simulink library "fbklib"  (R2015a)
settings: Solver=ode45  SolverMode=SingleTasking  StartTime=0.0  StopTime=10.0  RelTol=1e-3
settings Model: Creator=Fares  LastModifiedBy=Fares
settings DataIOCC: SignalLoggingSaveFormat=ModelDataLogs
settings OptimizationCC: BlockReduction=off  BooleanDataType=off
settings DebuggingCC: SaveWithParameterizedLinksMsg=none  UnderspecifiedInitializationDetection=Classic  MergeDetectMultiDrivingBlocksExec=none  SignalResolutionControl=TryResolveAllWithWarning  MultiTaskDSMMsg=warning  MultiTaskCondExecSysMsg=none  StrictBusMsg=None
settings HardwareCC: TargetUnknown=on

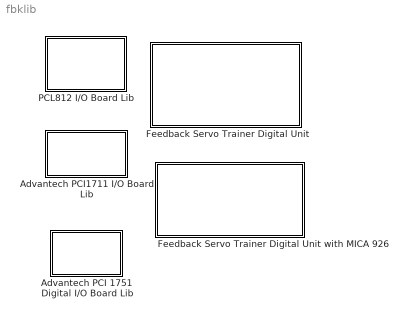
== system fbklib ==
  "Advantech PCI 1751 Digital I/O Board Lib " : Subsystem  AncestorBlock=|  mask(Advantech PCI 1751 Digital I/O Borad Lib.){}
      | pci1751/Advantech 
      | PCI 1751 Digital I//O
      | Board Lib
      mask Display: plot(0,0,100,100,[90,80,80,11,11],[90,90,20,20,80],[11,80],[80,80],[80,80],[20,14],[80,85,85,80],[45,45,66,66],[45,45,74,74],[20,13,13,20],[15,27,27,15,15],[75,75,26,26,75],[33,48,48,33,33],[75,75,55,55,75],[55,55,71,71,55],[55,75,75,55,55],[33,41,41,33,33],[50,50,27,27,50],[48,56,56,48,48],[50,50,27,27,50],[62,70,70,62,62],[50,50,27,27,50])
  Advantech PCI1711 I/O Board Lib : Subsystem  AncestorBlock="pci1711/Advantech  PCI1711 I//O Board Lib"  mask(PCI 1711 I/O Board Lib){}
      mask Display: plot(0,0,100,100,[90,80,80,11,11],[90,90,20,20,80],[11,80],[80,80],[80,80],[20,14],[80,85,85,80],[45,45,66,66],[45,45,74,74],[20,13,13,20],[15,27,27,15,15],[75,75,26,26,75],[33,48,48,33,33],[75,75,55,55,75],[55,55,71,71,55],[55,75,75,55,55],[33,41,41,33,33],[50,50,27,27,50],[48,56,56,48,48],[50,50,27,27,50],[62,70,70,62,62],[50,50,27,27,50])
  Feedback Servo Trainer Digital Unit : Subsystem  AncestorBlock=ServoTrainer/Feedback Servo Trainer Digital Unit  mask(Feedback Servo Trainer Digital Unit){}
      mask Display: disp ('Feedback 33-003 \n\n Digital Servo Fundementals ')
  Feedback Servo Trainer Digital Unit with MICA 926 : Subsystem  AncestorBlock=MicaServo/Feedback Servo Trainer Digital Unit  mask(Feedback Servo Trainer Digital Unit with Mica926){}
      mask Display: disp ('Feedback 33-003 \n\n Digital Servo Fundementals \n with MICA 926')
  PCL812 I/O Board Lib : Subsystem  AncestorBlock=Pcl812fbk/PCL812 I//O Board Lib  mask(PCL812 I/O Board Lib){}
      mask Display: plot(0,0,100,100,[90,80,80,11,11],[90,90,20,20,80],[11,80],[80,80],[80,80],[20,14],[80,85,85,80],[45,45,66,66],[45,45,74,74],[20,13,13,20],[15,27,27,15,15],[75,75,26,26,75],[33,48,48,33,33],[75,75,55,55,75],[55,55,71,71,55],[55,75,75,55,55],[33,41,41,33,33],[50,50,27,27,50],[48,56,56,48,48],[50,50,27,27,50],[62,70,70,62,62],[50,50,27,27,50])

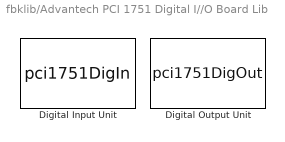
== system fbklib/Advantech PCI 1751 Digital I//O Board Lib  ==
  Digital Input Unit : S-Function  FunctionName=pci1751DigIn  Parameters=channel,portName,tsamp,hwaccess  mask(Digital Input Unit){channel=0, portName=A, tsamp=0.001, hwaccess=on}
      mask prompts: channel "Channel (0 or 1)"; portName "Input Port (A, B or  C)"; tsamp "sample Time (sec)"; hwaccess "Access Hardware"
      mask help: Digital Input Block for PCI1751
      mask Display: disp('PCI1751 \n Lab I/O Board \n\n Digital Input')
  Digital Output Unit : S-Function  FunctionName=pci1751DigOut  Parameters=channel,portName,tsamp,hwaccess  mask(Digital Output Unit){channel=0, portName=A, tsamp=0.001, hwaccess=on}
      mask prompts: channel "Channel (0 or 1)"; portName "Output Port (A, B, C or D)"; tsamp "sample Time (sec)"; hwaccess "Access Hardware"
      mask help: DigitalOutput Block for PCI1751
      mask Display: disp('PCI1751 \n Lab I/O Board \n\n Digital Output')

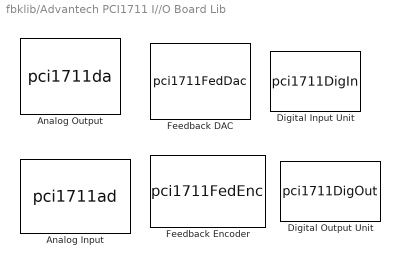
== system fbklib/Advantech PCI1711 I//O Board Lib ==
  Analog Input : S-Function  FunctionName=pci1711ad  Parameters=channel,rangeGain,tsamp,hwAccess  mask(Analog Input Unit){channel=0, rangeGain=0, tsamp=0.001, hwAccess=on}
      mask prompts: channel "Input Channel"; rangeGain "ADC Range Gain  (0 for -/+5V 1 for -/+2.5V 2 for -/+1.25 3 for -/+0.625V)"; tsamp "sampling Time (sec)"; hwAccess "Hardware Access"
      mask help:
      | Analog to Digital Input block for the
      |  Advantech PCI1711  I/O board
      mask Display: disp('PCI1711\n Lab I/O Board \n\n ADC')
  Analog Output : S-Function  FunctionName=pci1711da  Parameters=outChannel,range,tsamp,hwAccess  mask(Analog Output Unit){outChannel=0, range=0, tsamp=0.001, hwAccess=on}
      mask prompts: outChannel "Output Channel"; range "Range Selector (0 for 0-5V and 1 for 0-10V range)"; tsamp "sample Time (sec)"; hwAccess "Access Hardware"
      mask help:
      | Digital to Analog Output block for the
      |  Advantech PCI1711  I/O board
      mask Display: disp('PCI1711 \n Lab I/O Board \n\n DAC')
  Digital Input Unit : S-Function  FunctionName=pci1711DigIn  Parameters=channel,tsamp,hwaccess  mask(Digital Input Unit){channel=0, tsamp=0.001, hwaccess=on}
      mask prompts: channel "Channel (0 or 1)"; tsamp "sample Time (sec)"; hwaccess "Access Hardware"
      mask help: Digital Input Block
      mask Display: disp('PCI1711 \n Lab I/O Board \n\n Digital Input')
  Digital Output Unit : S-Function  FunctionName=pci1711DigOut  Parameters=channel,tsamp,hwAccess  mask(Digital Output Unit){channel=0, tsamp=0.001, hwAccess=on}
      mask prompts: channel "Channel (0 or 1)"; tsamp "sample Time (sec)"; hwAccess "Access Hardware"
      mask help: Digital Output Block
      mask Display: disp('PCI1711 \n Lab I/O Board \n\n Digital Output')
  Feedback DAC : S-Function  FunctionName=pci1711FedDac  Parameters=channel,range,tsamp,hwAccess  mask(DAC Unit for Feedback Experiments){channel=0, range=0, tsamp=0.001, hwAccess=on}
      mask prompts: channel "Output Channel"; range "Range Selector (0 for -/+2.5V, 1 for -/+5V range)"; tsamp "sample Time (sec)"; hwAccess "Access Hardware"
      mask help:
      | Digital to Analog Output  for Feedback Experiments
      | using Advantech PCI1711  I/O board
      mask Display: disp('PCI1711 \n Lab I/O Board \n\n Feedback  DAC')
  "Feedback Encoder " : S-Function  FunctionName=pci1711FedEnc  Parameters=channel,offset,tsamp,hwAccess  mask(Feedback Encoder Block){channel=0, offset=0, tsamp=0.001, hwAccess=on}
      mask prompts: channel "Channel (0 or 1)"; offset "Encoder Offset"; tsamp "sample Time (sec)"; hwAccess "Access Hardware"
      mask help: Special block to use with the Feedback experiments to read encoder channels using the digital I/O lines
      mask Display: disp('PCI1711 \n Lab I/O Board \n\n Feedback Encoder')

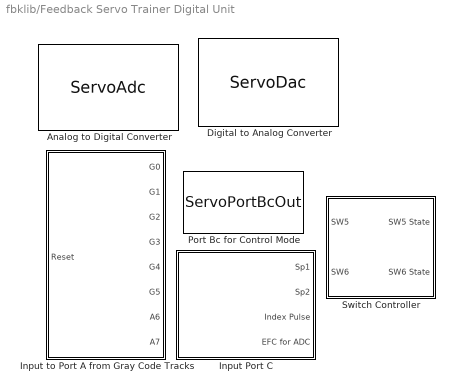
== system fbklib/Feedback Servo Trainer Digital Unit ==
  Analog to Digital Converter : S-Function  FunctionName=ServoAdc  Parameters=inType,stime, hwAccess  mask(Analog to Digital Converter){inType=RawData (-127 to +127), stime=0.01, hwAccess=on}
      mask prompts: inType "Input Type"; stime "Sampling Time (sec.)"; hwAccess "Access Hardware"
      mask help:
      | Analog Input Unit for Feedback DU154B
      | Digital Unit 33-003
      | Feeback Instruments
      mask Help:
      | Reads and converts the voltage applied to ADC input on the Digital Unit.
      | Read operation is done either in Rawdata (+/- 127) format or directly in voltage format
      mask TypeOptions inType: RawData (-127 to +127) |  Volt   (+/- 11V range)
      mask Display: disp('Feedback Servo Trainer\n Digital Unit 33-003\n\n ADC')
  Digital to Analog Converter : S-Function  FunctionName=ServoDac  Parameters=outType,stime, hwAccess  mask(Analog Output Module){outType=RawData (-127 to +127), stime=0.01, hwAccess=on}
      mask prompts: outType "Output Type :"; stime "Sampling Time (sec.)"; hwAccess "Access Hardware"
      mask help:
      | Analog Output Unit for Feedback DU154B
      | Digital Unit 33-003
      | Feeback Instruments
      mask Help:
      | Applies the corresponding voltage to the Servo Trainers DAC
      | output type can be selected to be either in RawData type or directly in volts
      mask TypeOptions outType: RawData (-127 to +127) |  Volt   (+/- 11V range)
      mask Display: disp('Feedback Servo Trainer\n Digital Unit 33-003\n\n DAC')
  Input Port C : Subsystem  mask(Read the Inputs from portC directly){stime=0.01, hwAccess=on}
      mask prompts: stime "Sample Time (sec.)"; hwAccess "Access Hardware"
  Input to Port A from Gray Code Tracks : Subsystem  mask(Read Gray Code and Speed Tracks){stime=0.01, hwAccess=on}
      mask prompts: stime "Sample Time (sec.)"; hwAccess "Hardware Access"
      mask help:
      | Read the inputs from the Gray Code tracks (A0-A5)
      | and Speed/Increment tracks (A6-A7)
      mask Help: no help is available for this block
  Port Bc for Control Mode : S-Function  FunctionName=ServoPortBcOut  Parameters=stime, hwAccess  mask(Port Bc for Direct access to Control Signals){stime=0.01, hwAccess=on}
      mask prompts: stime "Sample Time (sec.)"; hwAccess "Access Hardware"
      mask help:
      | To directly access the Bc control register
      | For Advanced users only !
      mask Help:
      | Will directly apply the integer input to the Bc control output
      | This module is for advenced users only .
      | using this module with other Servo Trainer modules may corrupt inputs !
      mask Display: disp('Feedback Servo Trainer\n Digital Unit 33-003\n\nPort Bc')
  Switch Controller : Subsystem  mask(Switch Controller){onWhen=1, stime=0.01, hwAccess=on}
      mask prompts: onWhen "Thresh Hold"; stime "Sample Time (sec.)"; hwAccess "Hardware Access"
      mask help:
      | Controls the SW5 and SW6 switches on the Digital Unit
      | The ouptut can be used to see the state of the switches
      mask Help: The Switches will be on when the input to the Swiches are bigger than or equal to the "Thresh Hold" variable

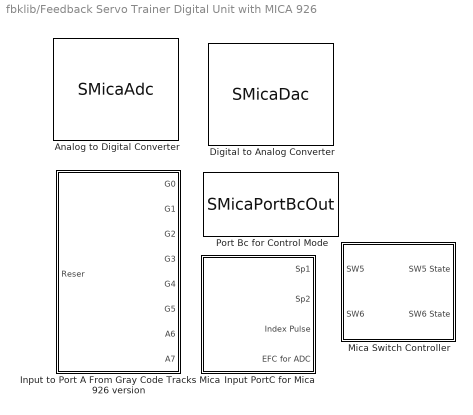
== system fbklib/Feedback Servo Trainer Digital Unit with MICA 926 ==
  " Digital to Analog Converter" : S-Function  FunctionName=SMicaDac  Parameters=baseAddr,inType,stime,hwAccess  mask(Digital to Analog Converter){baseAddr=0x300, inType=RawData (-127 to +127), stime=0.01, hwAccess=on}
      mask prompts: baseAddr "BaseAddress"; inType "Input Type"; stime "Sampling Time (sec.)"; hwAccess "Access Hardware"
      mask help:
      | Analog Input Unit for Feedback DU154B
      | Digital Unit 33-003
      | Feeback Instruments
      | MICA 926 Edition
      mask Help:
      | Applies the corresponding voltage to the Servo Trainers DAC
      | output type can be selected to be either in RawData type or directly in volts
      mask TypeOptions inType: RawData (-127 to +127) |  Volt   (+/- 11V range)
      mask Display: disp('Feedback Servo Trainer\n Digital Unit 33-003\n\n DAC\n Mica 926 Board ')
  Analog to Digital Converter : S-Function  FunctionName=SMicaAdc  Parameters=baseAddr,inType,stime,hwAccess  mask(Analog to Digital Converter){baseAddr=0x300, inType=RawData (-127 to +127), stime=0.01, hwAccess=on}
      mask prompts: baseAddr "BaseAddress"; inType "Input Type"; stime "Sampling Time (sec.)"; hwAccess "Access Hardware"
      mask help:
      | Analog Input Unit for Feedback DU154B
      | Digital Unit 33-003
      | Feeback Instruments
      mask Help:
      | Reads and converts the voltage applied to ADC input on the Digital Unit.
      | Read operation is done either in Rawdata (+/- 127) format or directly in voltage format
      mask TypeOptions inType: RawData (-127 to +127) |  Volt   (+/- 11V range)
      mask Display: disp('Feedback Servo Trainer\n Digital Unit 33-003\n\n ADC\n Mica 926 Board ')
  Input PortC for Mica : Subsystem  mask(Read the Inputs from portC directly){baseAddr=0x300, stime=0.01, hwAccess=on}
      mask prompts: baseAddr "BaseAddress"; stime "Sample Time (sec.)"; hwAccess "Access Hardware"
  Input to Port A From Gray Code Tracks Mica 926 version : Subsystem  mask(Read Gray Code and Speed Tracks){baseAddr=0x300, stime=0.01, hwAccess=on}
      mask prompts: baseAddr "BaseAddress"; stime "Sample Time (sec.)"; hwAccess "Hardware Access"
      mask help:
      | Read the inputs from the Gray Code tracks (A0-A5)
      | and Speed/Increment tracks (A6-A7)
      mask Help: no help is available for this block
  Mica Switch Controller : Subsystem  mask(Mica Switch Controller){baseAddr=0x300, onWhen=1.0, stime=0.01, hwAccess=on}
      mask prompts: baseAddr "BaseAddress"; onWhen "Thresh Hold"; stime "Sample Time (sec.)"; hwAccess "Hardware Access"
      mask help:
      | Controls the SW5 and SW6 switches on the Digital Unit
      | The ouptut can be used to see the state of the switches
      mask Help: The Switches will be on when the input to the Swiches are bigger than or equal to the "Thresh Hold" variable
  Port Bc for Control Mode : S-Function  FunctionName=SMicaPortBcOut  Parameters=baseAddr,stime,hwAccess  mask(Port Bc for Direct access to Control Signals){baseAddr=0x300, stime=0.01, hwAccess=on}
      mask prompts: baseAddr "Base Address"; stime "Sample Time (sec.)"; hwAccess "Access Hardware"
      mask help:
      | To directly access the Bc control register
      | For Advanced users only !
      mask Help:
      | Will directly apply the integer input to the Bc control output
      | This module is for advenced users only .
      | using this module with other Servo Trainer modules may corrupt inputs !
      mask Display: disp('Feedback Servo Trainer\n Digital Unit 33-003\n\nPort Bc \n Mica 926 Version')

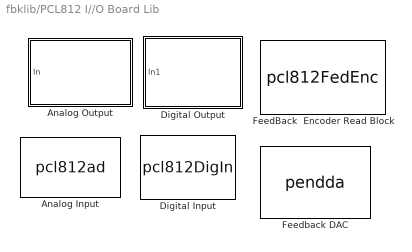
== system fbklib/PCL812 I//O Board Lib ==
  Analog Input : S-Function  FunctionName=pcl812ad  Parameters=baseAddr, inputChannel, AdcGain, AdcRange, stime,hwAcces  mask(Analog Output Module){baseAddr=0x220, inputChannel=0, AdcGain=1, AdcRange=5, stime=0.001, hwAcces=on}
      mask prompts: baseAddr "Base I/O Address :"; inputChannel "Input Channel :"; AdcGain "ADC Gain (1, 2, 4, 8, 16)"; AdcRange "ADC Range (either 5 or 10)"; stime "Sample Time (sec):"; hwAcces "Access Hardware"
      mask Display: disp('PCL812PG\n Lab I/O Board \n\n ADC')
  Analog Output : Subsystem  mask(Analog Output Module){baseAddr=0x220, outChannel=0, dacRef=5.0, stime=0.001, hwAcces=on}
      mask prompts: baseAddr "Base I/O Address:"; outChannel "Output Channel"; dacRef "Dac Reference Voltage"; stime "sample Time (sec):"; hwAcces "Access Hardware"
      mask help: Digital to Analog Output block for the PCL812 I/O board
      mask Help: no help is given for this block
      mask Display: disp('PCL812PG\n Lab I/O Board \n\n DAC')
  Digital Input : S-Function  FunctionName=pcl812DigIn  Parameters='0x220',0, 0.001, 1  mask(Digital Input Module){baseAddr=0x220, InByte=0, stime=0.001, hwAcces=on}
      mask prompts: baseAddr "Base I/O Address :"; InByte "Input Byte ('0' for Low '1' for High Byte)"; stime "Sample Time (sec)"; hwAcces "Acces Hardware"
      mask Display: disp('PCL812PG\n Lab I/O Board \n\n Digital Input')
  Digital Output : Subsystem  mask(Digital Output Model){baseAddr=0x220, outByte=0, stime=0.001, hwAcces=on}
      mask prompts: baseAddr "Base I/O Address:"; outByte "Output Byte ('0' for Low '1'  for High Byte)"; stime "Sample Time (sec):"; hwAcces "Acces Hardware"
      mask Display: disp('PCL812PG\n Lab I/O Board \n\n Digital Output')
  FeedBack  Encoder Read Block : S-Function  FunctionName=pcl812FedEnc  Parameters=baseAddr, Channel, stime ,encOffSet,hwAcces  mask(Encoder Module for FeedBack Experiments){baseAddr=0x220, Channel=1, stime=0.001, encOffSet=0, hwAcces=on}
      mask prompts: baseAddr "Base I/O Address :"; Channel "Channel (either 0 or 1)"; stime "sampling Time (sec) :"; encOffSet "Encoder Offset"; hwAcces "Access Hardware"
      mask help: Special block to use with the Feedback Experiments to read encoder signals using the digital IO lines
      mask Display: disp('PCL812PG\n Lab I/O Board \n\n FeedBackEncoder')
  Feedback DAC : S-Function  FunctionName=pendda  Parameters=baseAddr,outChannel, dacRef, stime, hwAcces  mask(DAC for Feebback Experiments){baseAddr=0x220, outChannel=1, dacRef=5, stime=0.001, hwAcces=on}
      mask prompts: baseAddr "Base I/O Address :"; outChannel "Output Channel"; dacRef "Dac Reference Voltage"; stime "Sample Time (sec):"; hwAcces "Access Hardware"
      mask Display: disp('PCL812PG\n Lab I/O Board \n\n FeedBack  DAC')

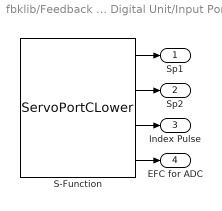
== system fbklib/Feedback Servo Trainer Digital Unit/Input Port C ==
  S-Function : S-Function  FunctionName=ServoPortCLower  Parameters=stime, hwAccess
  Sp1 : Outport
  Sp2 : Outport  Port=2
  Index Pulse : Outport  Port=3
  "EFC for ADC  " : Outport  Port=4
  wires:
  S-Function/4 -> "EFC for ADC  "/1
  S-Function/3 -> Index Pulse/1
  S-Function/2 -> Sp2/1
  S-Function/1 -> Sp1/1

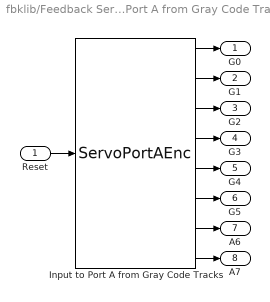
== system fbklib/Feedback Servo Trainer Digital Unit/Input to Port A from Gray Code Tracks ==
  Reset : Inport
  Input to Port A from Gray Code Tracks : S-Function  FunctionName=ServoPortAEnc  Parameters=stime,hwAccess
  G0 : Outport
  G1 : Outport  Port=2
  G2 : Outport  Port=3
  G3 : Outport  Port=4
  G4 : Outport  Port=5
  G5 : Outport  Port=6
  A6 : Outport  Port=7
  A7 : Outport  Port=8
  wires:
  Input to Port A from Gray Code Tracks/8 -> A7/1
  Input to Port A from Gray Code Tracks/7 -> A6/1
  Input to Port A from Gray Code Tracks/6 -> G5/1
  Input to Port A from Gray Code Tracks/5 -> G4/1
  Reset/1 -> Input to Port A from Gray Code Tracks/1
  Input to Port A from Gray Code Tracks/4 -> G3/1
  Input to Port A from Gray Code Tracks/3 -> G2/1
  Input to Port A from Gray Code Tracks/2 -> G1/1
  Input to Port A from Gray Code Tracks/1 -> G0/1

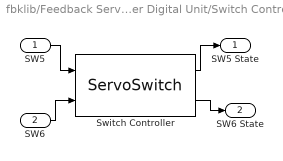
== system fbklib/Feedback Servo Trainer Digital Unit/Switch Controller ==
  SW5 : Inport
  SW6 : Inport  Port=2
  Switch Controller : S-Function  FunctionName=ServoSwitch  Parameters=onWhen,stime, hwAccess
  SW5 State : Outport
  SW6 State : Outport  Port=2
  wires:
  SW6/1 -> Switch Controller/2
  Switch Controller/2 -> SW6 State/1
  SW5/1 -> Switch Controller/1
  Switch Controller/1 -> SW5 State/1

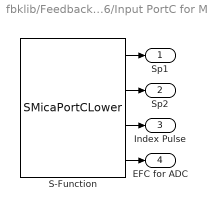
== system fbklib/Feedback Servo Trainer Digital Unit with MICA 926/Input PortC for Mica ==
  S-Function : S-Function  FunctionName=SMicaPortCLower  Parameters=baseAddr,stime,hwAccess
  Sp1 : Outport
  Sp2 : Outport  Port=2
  Index Pulse : Outport  Port=3
  "EFC for ADC  " : Outport  Port=4
  wires:
  S-Function/1 -> Sp1/1
  S-Function/2 -> Sp2/1
  S-Function/3 -> Index Pulse/1
  S-Function/4 -> "EFC for ADC  "/1

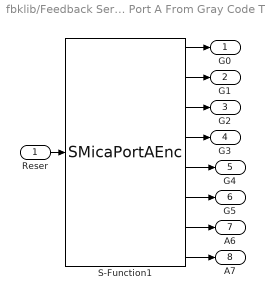
== system fbklib/Feedback Servo Trainer Digital Unit with MICA 926/Input to Port A From Gray Code Tracks Mica 926 version ==
  Reser : Inport
  S-Function1 : S-Function  FunctionName=SMicaPortAEnc  Parameters=baseAddr,stime,hwAccess
  G0 : Outport
  G1 : Outport  Port=2
  G2 : Outport  Port=3
  G3 : Outport  Port=4
  G4 : Outport  Port=5
  G5 : Outport  Port=6
  A6 : Outport  Port=7
  A7 : Outport  Port=8
  wires:
  S-Function1/1 -> G0/1
  S-Function1/2 -> G1/1
  S-Function1/3 -> G2/1
  S-Function1/4 -> G3/1
  Reser/1 -> S-Function1/1
  S-Function1/5 -> G4/1
  S-Function1/6 -> G5/1
  S-Function1/7 -> A6/1
  S-Function1/8 -> A7/1

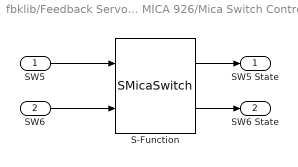
== system fbklib/Feedback Servo Trainer Digital Unit with MICA 926/Mica Switch Controller ==
  SW5 : Inport
  SW6 : Inport  Port=2
  S-Function : S-Function  FunctionName=SMicaSwitch  Parameters=baseAddr,onWhen,stime,hwAccess
  SW5 State : Outport
  SW6 State : Outport  Port=2
  wires:
  S-Function/1 -> SW5 State/1
  SW5/1 -> S-Function/1
  S-Function/2 -> SW6 State/1
  SW6/1 -> S-Function/2

== system fbklib/PCL812 I//O Board Lib/Analog Output ==
  In : Inport
  S-Function : S-Function  FunctionName=pcl812da  Parameters=baseAddr,outChannel, dacRef, stime, hwAcces
  wires:
  In/1 -> S-Function/1

== system fbklib/PCL812 I//O Board Lib/Digital Output ==
  In1 : Inport
  S-Function : S-Function  FunctionName=pcl812DigOut  Parameters=baseAddr,outByte, stime, hwAcces
  wires:
  In1/1 -> S-Function/1
